simulink model "positionCalculateSimulate"  (R2022b)
settings: Solver=VariableStepAuto  StartTime=0.0  StopTime=20  RelTol=1e-3
settings Model: Creator=96234  LastModifiedBy=96234

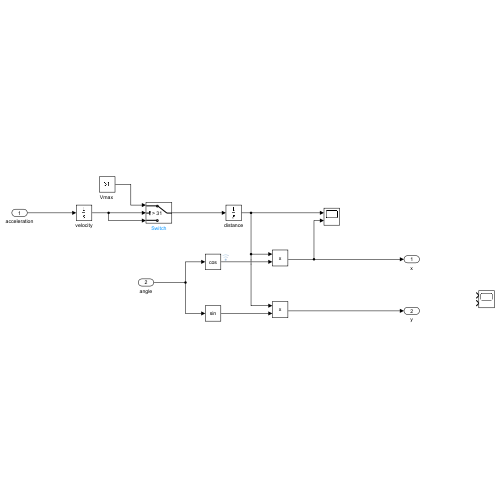
[thumbnail: Simulink's stored preview of the top-level diagram]
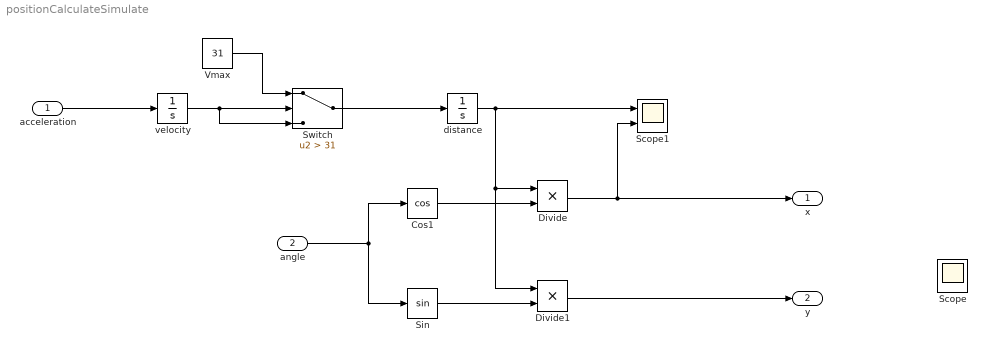
== system positionCalculateSimulate ==
  acceleration : Inport
  angle : Inport  Port=2
  Cos1 : Trigonometry  Operator=cos
  Divide : Product  Inputs=**
  Divide1 : Product  Inputs=**
  Scope : Scope  NumInputPorts=2
  Scope1 : Scope  NumInputPorts=2
  Sin : Trigonometry
  Switch : Switch  Criteria=u2 > Threshold  Threshold=31  SaturateOnIntegerOverflow=off  InputSameDT=off
  "Vmax " : Constant  Value=31
  distance : Integrator
  velocity : Integrator
  x : Outport
  y : Outport  Port=2
  wires:
  acceleration/1 -> velocity/1
  velocity/1 -> Switch/3, Switch/2
  "Vmax "/1 -> Switch/1
  Switch/1 -> distance/1
  distance/1 -> Scope1/1, Divide1/1, Divide/1
  Cos1/1 -> Divide/2
  Divide/1 -> Scope1/2, x/1
  angle/1 -> Sin/1, Cos1/1
  Sin/1 -> Divide1/2
  Divide1/1 -> y/1
